simulink model "mpc_control_casadi_c_implement"  (R2022b)
settings: Solver=VariableStepAuto  StartTime=0.0  StopTime=20  RelTol=1e-3
libraries: Solver_SF x1, slpidlib x1
settings Model: Creator=Miakho  LastModifiedBy=Miakho

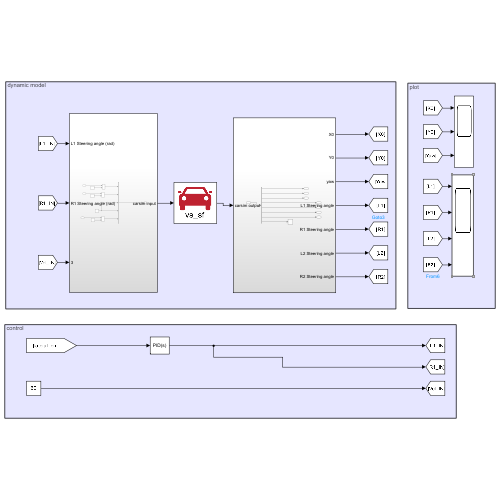
[thumbnail: Simulink's stored preview of the top-level diagram]
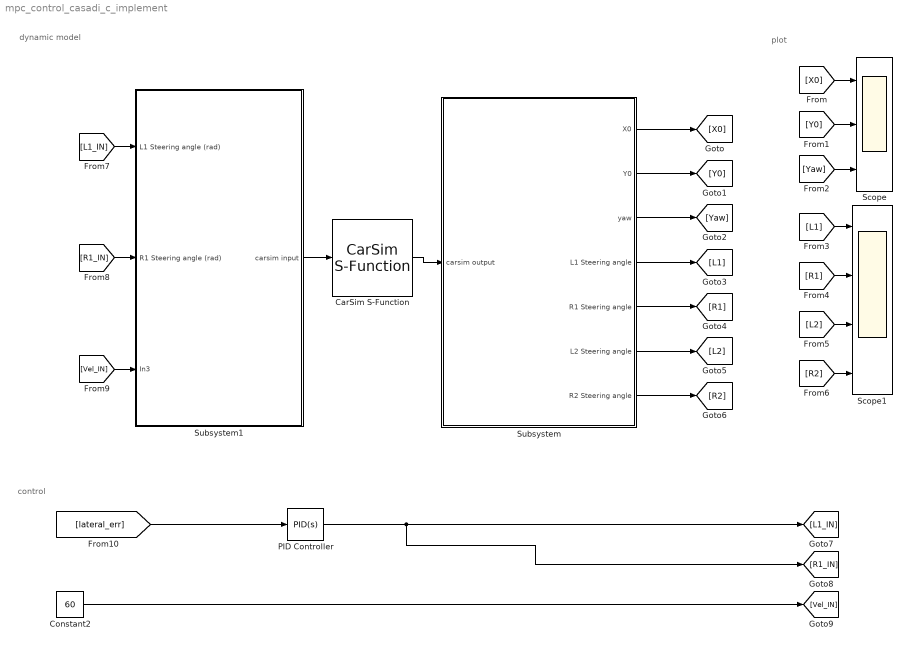
== system mpc_control_casadi_c_implement ==
  note: control
  note: dynamic model
  note: plot
  CarSim S-Function : Solver_SF/CarSim S-Function  Priority=1  SIMFILE=simfile.sim  Run_RTs=off  vs_state_ind=Run  StopMode_ind=Vehicle Model
  Constant2 : Constant  Value=60
  PID Controller : slpidlib/PID Controller  Controller=PID  Form=Parallel  TimeDomain=Continuous-time  UseExternalTs=off  SampleTime=-1  IntegratorMethod=Forward Euler  FilterMethod=Forward Euler  ControllerParametersSource=internal  P=4  I=0  UseKiTs=off  D=1  N=100  UseFilter=on  TunerSelectOption=Transfer Function Based (PID Tuner App)  InitialConditionSource=internal  InitialConditionForIntegrator=0  InitialConditionForFilter=0  DifferentiatorICPrevScaledInput=0  ExternalReset=none  TrackingMode=off  Kt=1  LimitOutput=off  SatLimitsSource=internal  UpperSaturationLimit=inf  LowerSaturationLimit=-inf  LinearizeAsGain=on  AntiWindupMode=none  Kb=1  LimitIntegrator=off  UpperIntegratorSaturationLimit=inf  LowerIntegratorSaturationLimit=-inf  POutMin=[]  POutMax=[]  IOutMin=[]  IOutMax=[]  DOutMin=[]  DOutMax=[]  NOutMin=[]  NOutMax=[]  SumOutMin=[]  SumOutMax=[]  SaturationOutMin=[]  SaturationOutMax=[]  PParamMin=[]  PParamMax=[]  IParamMin=[]  IParamMax=[]  DParamMin=[]  DParamMax=[]  NParamMin=[]  NParamMax=[]  KbParamMin=[]  KbParamMax=[]  KtParamMin=[]  KtParamMax=[]  KbOutMin=[]  KbOutMax=[]  KtOutMin=[]  KtOutMax=[]  IntegratorOutMin=[]  IntegratorOutMax=[]  FilterOutMin=[]  FilterOutMax=[]  SumI1OutMin=[]  SumI1OutMax=[]  SumI2OutMin=[]  SumI2OutMax=[]  SumI3OutMin=[]  SumI3OutMax=[]  SumI4OutMin=[]  SumI4OutMax=[]  SumDOutMin=[]  SumDOutMax=[]  DifferentiatorOutMin=[]  DifferentiatorOutMax=[]  FilterDiffOutCoefMin=[]  FilterDiffOutCoefMax=[]  ReciprocalOutMin=[]  ReciprocalOutMax=[]  SumDenOutMin=[]  SumDenOutMax=[]  SumNumOutMin=[]  SumNumOutMax=[]  DivideOutMin=[]  DivideOutMax=[]  UdiffTsProdOutMin=[]  UdiffTsProdOutMax=[]  NTsProdOutMin=[]  NTsProdOutMax=[]  UintegralTsProdOutMin=[]  UintegralTsProdOutMax=[]  UngainTsProdOutMin=[]  UngainTsProdOutMax=[]  ClampingZeroOutDataTypeStr=Inherit: Inherit via back propagation  ClampingZeroOutMin=[]  ClampingZeroOutMax=[]  FilterDenConstantOutDataTypeStr=Inherit: Inherit via back propagation  FilterDenConstantOutMin=[]  FilterDenConstantOutMax=[]  PCopyOutDataTypeStr=Inherit: Inherit via back propagation  PCopyOutMin=[]  PCopyOutMax=[]  NCopyOutDataTypeStr=Inherit: Inherit via back propagation  NCopyOutMin=[]  NCopyOutMax=[]  IntegratorContinuousStateAttributes=''  IntegratorStateMustResolveToSignalObject=off  IntegratorRTWStateStorageClass=Auto  FilterContinuousStateAttributes=''  FilterStateMustResolveToSignalObject=off  FilterRTWStateStorageClass=Auto  ParallelPVariant=InternalParameters  IdealPVariant=Disabled  IVariant=InternalParameters  DVariant=InternalParameters  IntegratorVariant=Continuous  SatVariant=Disabled  AWVariant=Passthrough  PCopyVariant=Disabled  TRVariant=Disabled  FdbkBlocksVariant=Forward  IdealPFdbkVariant=Disabled  SatFdbkVariant=Disabled  DerivativeFilterVariant=ContFilter  NVariant=InternalParameters  NCopyVariant=Disabled  FilterICVariant=InternalICsFilter  IntegratorICVariant=InternalICs  ExternalResetVariant=Disabled  TRSumVariant=Passthrough  SumFdbkVariant=Disabled  SumVariant=Sum_PID  TsampFilterVariant=InternalTs  TsampNgainVariant=Passthrough  TsampIntegralVariant=Passthrough  ExternalSaturationOutDataTypeStr=Inherit: Same as second input
  Scope : Scope  NumInputPorts=3
  Scope1 : Scope  NumInputPorts=4
  Subsystem : Subsystem
  Subsystem1 : Subsystem
  wires:
  CarSim S-Function/1 -> Subsystem/1(carsim output)
  Subsystem/3(yaw) -> [Yaw]
  Subsystem/4(L1 Steering angle) -> [L1]
  Subsystem1/1(carsim input) -> CarSim S-Function/1
  Subsystem/1(X0) -> [X0]
  [X0] -> Scope/1
  Subsystem/2(Y0) -> [Y0]
  [Y0] -> Scope/2
  [Yaw] -> Scope/3
  [L1] -> Scope1/1
  Subsystem/5(R1 Steering angle) -> [R1]
  [R1] -> Scope1/2
  Subsystem/6(L2 Steering angle) -> [L2]
  [L2] -> Scope1/3
  Subsystem/7(R2 Steering angle) -> [R2]
  [R2] -> Scope1/4
  PID Controller/1 -> [R1_IN], [L1_IN]
  [L1_IN] -> Subsystem1/1(L1 Steering angle (rad))
  [R1_IN] -> Subsystem1/2(R1 Steering angle (rad))
  Constant2/1 -> [Vel_IN]
  [Vel_IN] -> Subsystem1/3(In3)
  [lateral_err] -> PID Controller/1

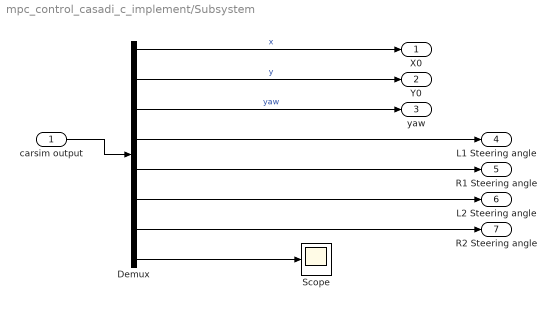
== system mpc_control_casadi_c_implement/Subsystem ==
  carsim output : Inport
  Demux : Demux  Outputs=8
  Scope : Scope
  X0 : Outport
  Y0 : Outport  Port=2
  yaw : Outport  Port=3
  L1 Steering angle : Outport  Port=4
  R1 Steering angle : Outport  Port=5
  L2 Steering angle : Outport  Port=6
  R2 Steering angle : Outport  Port=7
  wires:
  Demux/3 -> yaw/1  "yaw"
  Demux/1 -> X0/1  "x"
  carsim output/1 -> Demux/1
  Demux/6 -> L2 Steering angle/1
  Demux/7 -> R2 Steering angle/1
  Demux/4 -> L1 Steering angle/1
  Demux/2 -> Y0/1  "y"
  Demux/5 -> R1 Steering angle/1
  Demux/8 -> Scope/1

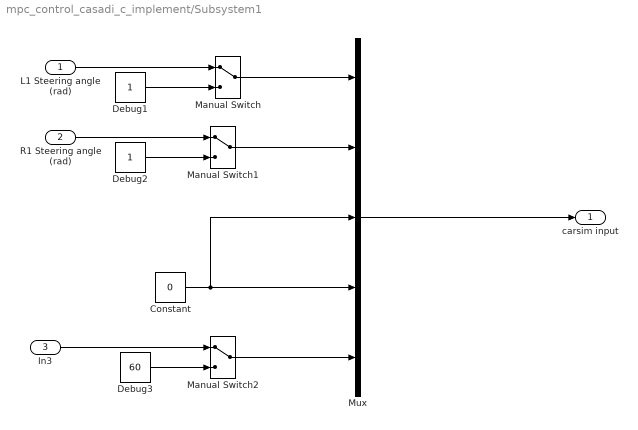
== system mpc_control_casadi_c_implement/Subsystem1 ==
  L1 Steering angle (rad) : Inport
  R1 Steering angle (rad) : Inport  Port=2
  In3 : Inport  Port=3
  Constant : Constant  Value=0
  Debug1 : Constant
  Debug2 : Constant
  Debug3 : Constant  Value=60
  Manual Switch : ManualSwitch
  Manual Switch1 : ManualSwitch
  Manual Switch2 : ManualSwitch
  Mux : Mux  Inputs=5
  carsim input : Outport
  wires:
  R1 Steering angle (rad)/1 -> Manual Switch1/1
  Mux/1 -> carsim input/1
  In3/1 -> Manual Switch2/1
  L1 Steering angle (rad)/1 -> Manual Switch/1
  Constant/1 -> Mux/3, Mux/4
  Debug1/1 -> Manual Switch/2
  Manual Switch/1 -> Mux/1
  Manual Switch1/1 -> Mux/2
  Debug2/1 -> Manual Switch1/2
  Debug3/1 -> Manual Switch2/2
  Manual Switch2/1 -> Mux/5
